simulink model "test_to_delete"  (R2019b)
settings: Solver=VariableStepAuto  StartTime=0.0  StopTime=10.0  MaxStep=0.1  MinStep=0.1  RelTol=1e-3
settings Model: Creator=maxim  LastModifiedBy=maxim
settings SolverCC: InitialStep=0.1

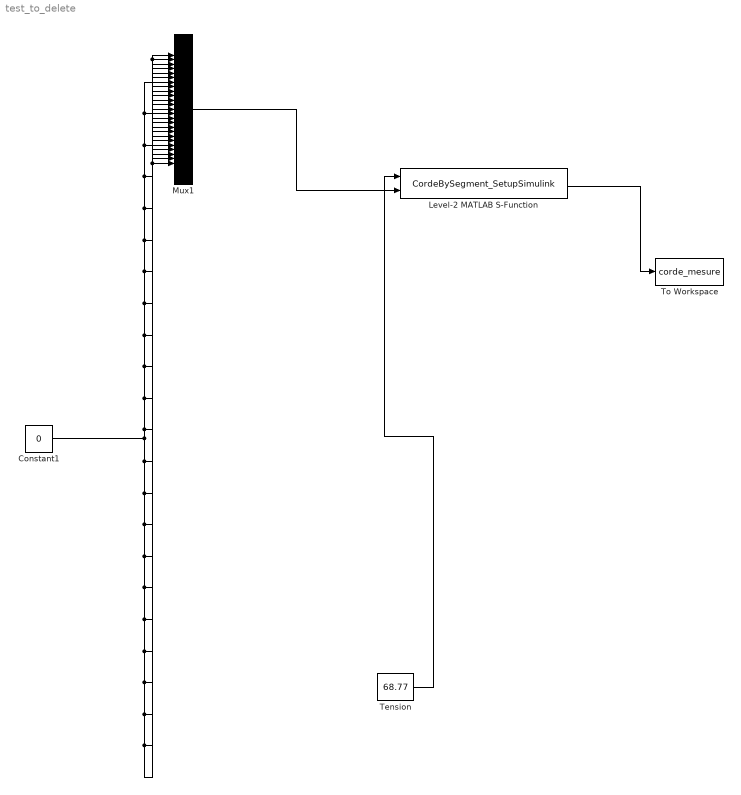
== system test_to_delete ==
  Constant1 : Constant  Value=0
  Level-2 MATLAB S-Function : M-S-Function  FunctionName=CordeBySegment_SetupSimulink  Parameters=0.00325,0.443,0,25
  Mux1 : Mux  Inputs=25
  "Tension " : Constant  Value=68.77
  To Workspace : ToWorkspace  VariableName=corde_mesure  SaveFormat=Timeseries  SampleTime=-1
  wires:
  Level-2 MATLAB S-Function/1 -> To Workspace/1
  "Tension "/1 -> Level-2 MATLAB S-Function/1
  Constant1/1 -> Mux1/25, Mux1/24, Mux1/23, Mux1/22, Mux1/21, Mux1/20, Mux1/19, Mux1/18, Mux1/17, Mux1/16, Mux1/15, Mux1/14, Mux1/1, Mux1/2, Mux1/3, Mux1/4, Mux1/5, Mux1/6, Mux1/7, Mux1/8, Mux1/9, Mux1/10, Mux1/11, Mux1/12, Mux1/13
  Mux1/1 -> Level-2 MATLAB S-Function/2
